simulink model "vector_testing"  (R2021a)
settings: Solver=VariableStepAuto  StartTime=0.0  StopTime=10.0  RelTol=1e-3
libraries: hdlBasic x18, hdlSSR x6, xbsIndex_r4 x1
settings Model: Creator=ckk5  LastModifiedBy=ckk5

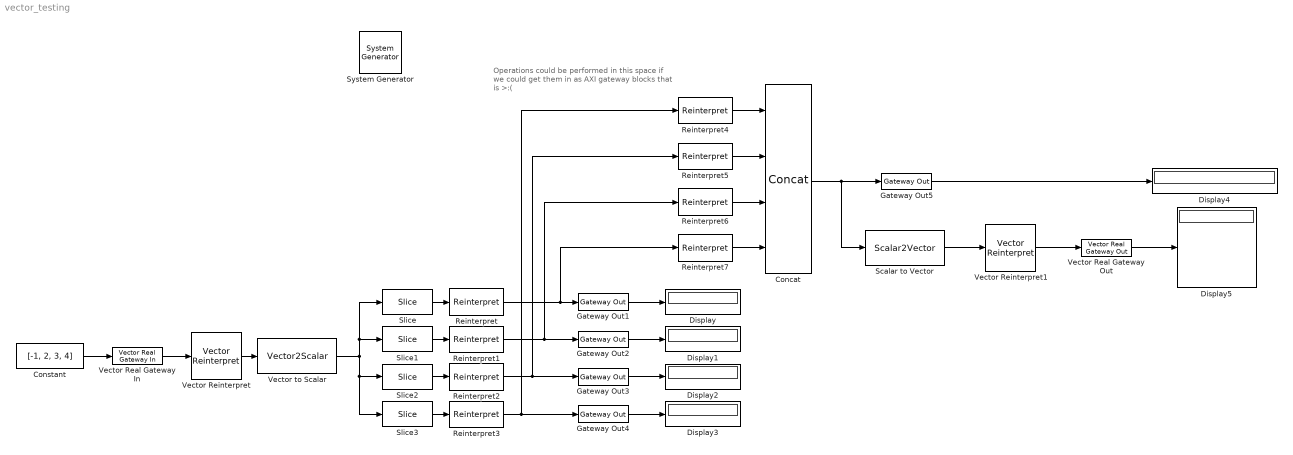
== system vector_testing ==
  note: Operations could be performed in this space
      | if we could get them in as AXI gateway blocks
      | that is >:(
  " System Generator" : xbsIndex_r4/ System Generator  Tag=genX  xilinxfamily=zynq  part=xc7z020  speed=-1  package=clg484  synthesis_tool=Vivado  clock_wrapper=Clock Enables  directory=./netlist  proj_type=Vivado  Synth_file=Vivado Synthesis Defaults  Impl_file=Vivado Implementation Defaults  testbench=off  simulink_period=1/4  sysclk_period=10  dcm_input_clock_period=10  incr_netlist=off  trim_vbits=Everywhere in SubSystem  dbl_ovrd=According to Block Masks  core_generation=According to Block Masks  run_coregen=off  deprecated_control=off  eval_field=0  block_type=sysgen
  Concat : hdlBasic/Concat  num_inputs=4  XmcBlockStatus=1  maskContainerNames=group1  block_type=concat  block_config=sysgen:Concat_config
  Constant : Constant  Value=[-1, 2, 3, 4]
  Display{,1..5} (6 alike) : Display
      Display settings: Format=hex (Stored Integer)
      Display1 settings: Format=binary (Stored Integer)
      Display2 settings: Format=binary (Stored Integer)
      Display3 settings: Format=binary (Stored Integer)
      Display4 settings: Format=hex (Stored Integer)
      Display5 settings: Format=hex (Stored Integer)
  Gateway Out{1..5} (5 alike) : hdlBasic/Gateway Out  inherit_from_input=off  hdl_port=off  rows=1  columns=1  UseAsDAC=off  DACChannel='1'  interface=None  automatic_assignment=on  address_offset=hex2dec('00')  intf_name=''  intf_description=''  timing_constraint=None  locs_specified=off  LOCs={}  io_standard={}  XmcBlockStatus=1  maskContainerNames=group4  block_type=gatewayout  block_config=sysgen:gateway_out_config  block_width_w=590  block_height_w=620  block_width=620  block_height=750
  Reinterpret{,1..3} (4 alike) : hdlBasic/Reinterpret  force_arith_type=on  arith_type="Signed  (2's comp)"  force_bin_pt=on  bin_pt=12  XmcBlockStatus=1  maskContainerNames=group1  block_type=reinterpret  block_config=sysgen:Reinterpret_config
  Reinterpret{4..7} (4 alike) : hdlBasic/Reinterpret  force_arith_type=on  arith_type=Unsigned  force_bin_pt=on  bin_pt=0  XmcBlockStatus=1  maskContainerNames=group1  block_type=reinterpret  block_config=sysgen:Reinterpret_config
  Scalar to Vector : hdlSSR/Scalar2Vector  Width=16  sg_ssr=4  block_type=scalar2vector_ssr  XmcBlockStatus=1  sg_ssr_prev=4  maskContainerNames=group1
  Slice : hdlBasic/Slice  nbits=16  boolean_output=off  mode=Lower Bit Location + Width  bit1=0  base1=LSB of Input  bit0=0  base0=LSB of Input  XmcBlockStatus=1  maskContainerNames=group1  block_type=slice  block_config=sysgen:Slice_config
  Slice1 : hdlBasic/Slice  nbits=16  boolean_output=off  mode=Lower Bit Location + Width  bit1=17  base1=LSB of Input  bit0=16  base0=LSB of Input  XmcBlockStatus=1  maskContainerNames=group1  block_type=slice  block_config=sysgen:Slice_config
  Slice2 : hdlBasic/Slice  nbits=16  boolean_output=off  mode=Lower Bit Location + Width  bit1=33  base1=LSB of Input  bit0=32  base0=LSB of Input  XmcBlockStatus=1  maskContainerNames=group1  block_type=slice  block_config=sysgen:Slice_config
  Slice3 : hdlBasic/Slice  nbits=16  boolean_output=off  mode=Lower Bit Location + Width  bit1=49  base1=LSB of Input  bit0=48  base0=LSB of Input  XmcBlockStatus=1  maskContainerNames=group1  block_type=slice  block_config=sysgen:Slice_config
  Vector Real Gateway In : hdlSSR/Vector Real Gateway In  gui_display_data_type=Fixed-point  arith_type=Signed (2's comp)  n_bits=16  bin_pt=12  preci_type=Single  exp_width=8  frac_width=24  quantization="Round  (unbiased: +/- Inf)"  overflow=Saturate  period=1  sg_ssr=4  UseAsADC=off  ADCChannel='1'  interface=None  automatic_assignment=on  address_offset=hex2dec('00')  intf_name=''  intf_description=''  default_value=0  timing_constraint=None  locs_specified=off  LOCs={}  io_standard={}  inherit_from_input=off  hdl_port=on  interface_prev=1  block_type=realgatewayin_ssr  XmcBlockStatus=1  sg_ssr_prev=4  maskContainerNames=group4  block_width_w=590  block_height_w=670  block_width=640  block_height=850
  Vector Real Gateway Out : hdlSSR/Vector Real Gateway Out  inherit_from_input=off  hdl_port=on  sg_ssr=4  rows=1  columns=1  UseAsDAC=off  DACChannel='1'  interface=None  automatic_assignment=on  address_offset=hex2dec('00')  intf_name=''  intf_description=''  timing_constraint=None  locs_specified=off  LOCs={}  io_standard={}  block_type=realgatewayout_ssr  XmcBlockStatus=1  sg_ssr_prev=4  maskContainerNames=group4  block_width_w=590  block_height_w=620  block_width=620  block_height=750
  Vector Reinterpret : hdlSSR/Vector Reinterpret  force_arith_type=on  arith_type=Unsigned  force_bin_pt=on  bin_pt=0  sg_ssr=4  block_type=reinterpret_ssr  XmcBlockStatus=1  sg_ssr_prev=4  maskContainerNames=group1
  Vector Reinterpret1 : hdlSSR/Vector Reinterpret  force_arith_type=on  arith_type="Signed  (2's comp)"  force_bin_pt=on  bin_pt=12  sg_ssr=4  block_type=reinterpret_ssr  XmcBlockStatus=1  sg_ssr_prev=4  maskContainerNames=group1
  Vector to Scalar : hdlSSR/Vector2Scalar  sg_ssr=4  block_type=vector2scalar_ssr  XmcBlockStatus=1  sg_ssr_prev=4  maskContainerNames=group1
  wires:
  Vector to Scalar/1 -> Slice/1, Slice1/1, Slice3/1, Slice2/1
  Slice3/1 -> Reinterpret3/1
  Slice2/1 -> Reinterpret2/1
  Slice1/1 -> Reinterpret1/1
  Slice/1 -> Reinterpret/1
  Gateway Out1/1 -> Display/1
  Gateway Out2/1 -> Display1/1
  Gateway Out3/1 -> Display2/1
  Gateway Out4/1 -> Display3/1
  Gateway Out5/1 -> Display4/1
  Scalar to Vector/1 -> Vector Reinterpret1/1
  Vector Real Gateway Out/1 -> Display5/1
  Concat/1 -> Scalar to Vector/1, Gateway Out5/1
  Vector Reinterpret/1 -> Vector to Scalar/1
  Vector Reinterpret1/1 -> Vector Real Gateway Out/1
  Vector Real Gateway In/1 -> Vector Reinterpret/1
  Constant/1 -> Vector Real Gateway In/1
  Reinterpret/1 -> Reinterpret7/1, Gateway Out1/1
  Reinterpret1/1 -> Reinterpret6/1, Gateway Out2/1
  Reinterpret2/1 -> Reinterpret5/1, Gateway Out3/1
  Reinterpret3/1 -> Reinterpret4/1, Gateway Out4/1
  Reinterpret4/1 -> Concat/1
  Reinterpret5/1 -> Concat/2
  Reinterpret6/1 -> Concat/3
  Reinterpret7/1 -> Concat/4
